simulink model "npc_controller"  (R2022a)
settings: Solver=FixedStepDiscrete  StartTime=0.0  StopTime=20  RelTol=1e-3  EnableMultiTasking=on
undefined symbols (not defined in the file): CAN_O_INT, CANA_BASE, Down, GPTRIP1SEL, GPTRIP2SEL, GPTRIP3SEL, Tsw, TZ1, TZ2, TZ3, Up
libraries: simulink x147, hdlsllib x90, c2802xlib x34, c2837xDlib x20, c280xlib x12, canmsglib x9, c2838xlib x8, idelinklib_common x3, c2806xlib x2, slpidlib x2, c28004xlib x2, c281xlib x2
(part 29 of 42)

== system npc_controller/IDLE_AND_TIMER/codegen/IDLE/idle_task/report_status_flag_bits ==
  Action Port : ActionPort  ActionPortLabel=case [ 0 ]:
  Add : Sum  Inputs=+++++++++++++
  Bit Shift1 : hdlsllib/Logic and Bit Operations/Bit Shift  mode=Shift Left Logical  N=4
  Bit Shift10 : hdlsllib/Logic and Bit Operations/Bit Shift  mode=Shift Left Logical  N=13
  Bit Shift11 : hdlsllib/Logic and Bit Operations/Bit Shift  mode=Shift Left Logical  N=14
  Bit Shift12 : hdlsllib/Logic and Bit Operations/Bit Shift  mode=Shift Left Logical  N=15
  Bit Shift2 : hdlsllib/Logic and Bit Operations/Bit Shift  mode=Shift Left Logical  N=5
  Bit Shift3 : hdlsllib/Logic and Bit Operations/Bit Shift  mode=Shift Left Logical  N=6
  Bit Shift4 : hdlsllib/Logic and Bit Operations/Bit Shift  mode=Shift Left Logical  N=8
  Bit Shift5 : hdlsllib/Logic and Bit Operations/Bit Shift  mode=Shift Left Logical  N=9
  Bit Shift6 : hdlsllib/Logic and Bit Operations/Bit Shift  mode=Shift Left Logical  N=7
  Bit Shift7 : hdlsllib/Logic and Bit Operations/Bit Shift  mode=Shift Left Logical  N=10
  Bit Shift8 : hdlsllib/Logic and Bit Operations/Bit Shift  mode=Shift Left Logical  N=11
  Bit Shift9 : hdlsllib/Logic and Bit Operations/Bit Shift  mode=Shift Left Logical  N=12
  Data Store Read1 : DataStoreRead  DataStoreName=pos_seq  IndexOptions=Index vector (dialog)  Indices=1  OutputSizes=1
  Data Store Read10 : DataStoreRead  DataStoreName=pfc_en  IndexOptions=Index vector (dialog)  Indices=1  OutputSizes=1
  Data Store Read12 : DataStoreRead  DataStoreName=rec_en  IndexOptions=Index vector (dialog)  Indices=1  OutputSizes=1
  Data Store Read13 : DataStoreRead  DataStoreName=ac_ok  IndexOptions=Index vector (dialog)  Indices=1  OutputSizes=1
  Data Store Read14 : DataStoreRead  DataStoreName=can_on_cmd  IndexOptions=Index vector (dialog)  Indices=1  OutputSizes=1
  Data Store Read2 : DataStoreRead  DataStoreName=clllc_ok  IndexOptions=Index vector (dialog)  Indices=1  OutputSizes=1
  Data Store Read3 : DataStoreRead  DataStoreName=npc_fault  IndexOptions=Index vector (dialog)  Indices=1  OutputSizes=1
  Data Store Read4 : DataStoreRead  DataStoreName=inv_en  IndexOptions=Index vector (dialog)  Indices=1  OutputSizes=1
  Data Store Read5 : DataStoreRead  DataStoreName=pfc_ok  IndexOptions=Index vector (dialog)  Indices=1  OutputSizes=1
  Data Store Read6 : DataStoreRead  DataStoreName=state_control  IndexOptions=Index vector (dialog)  Indices=1  OutputSizes=1
  Data Store Read7 : DataStoreRead  DataStoreName=relay_ctrl  IndexOptions=Index vector (dialog)  Indices=1  OutputSizes=1
  Data Store Read8 : DataStoreRead  DataStoreName=ot_fault  IndexOptions=Index vector (dialog)  Indices=1  OutputSizes=1
  Data Store Read9 : DataStoreRead  DataStoreName=can_timeout  IndexOptions=Index vector (dialog)  Indices=1  OutputSizes=1
  Data Store Write : DataStoreWrite  DataStoreName=sPriStatus  IndexOptions=Index vector (dialog)  Indices=1  OutputSizes=1
  Data Store Write4 : DataStoreWrite  Commented=on  DataStoreName=u8ThermalFlags  IndexOptions=Index vector (dialog)  Indices=1  OutputSizes=1
  Data Store Write5 : DataStoreWrite  Commented=on  DataStoreName=u8Reserved1  IndexOptions=Index vector (dialog)  Indices=1  OutputSizes=1
  Data Store Write6 : DataStoreWrite  Commented=on  DataStoreName=u16Reserved1  IndexOptions=Index vector (dialog)  Indices=1  OutputSizes=1
  Data Type Conversion{,1..12} (13 alike) : DataTypeConversion  OutDataTypeStr=uint16  SaturateOnIntegerOverflow=off  RndMeth=Floor
  wires:
  Bit Shift9/1 -> Add/10
  Data Store Read8/1 -> Data Type Conversion11/1
  Data Type Conversion10/1 -> Bit Shift10/1
  Data Type Conversion2/1 -> Bit Shift2/1
  Data Store Read1/1 -> Data Type Conversion5/1
  Bit Shift5/1 -> Add/7
  Data Type Conversion9/1 -> Bit Shift9/1
  Data Type Conversion12/1 -> Bit Shift12/1
  Data Store Read6/1 -> Data Type Conversion/1
  Add/1 -> Data Store Write/1
  Data Store Read9/1 -> Data Type Conversion12/1
  Data Store Read7/1 -> Data Type Conversion6/1
  Bit Shift7/1 -> Add/8
  Data Type Conversion/1 -> Add/1
  Data Type Conversion1/1 -> Bit Shift1/1
  Data Type Conversion8/1 -> Bit Shift8/1
  Bit Shift4/1 -> Add/6
  Data Store Read5/1 -> Data Type Conversion8/1
  Bit Shift3/1 -> Add/4
  Data Type Conversion11/1 -> Bit Shift11/1
  Data Type Conversion3/1 -> Bit Shift3/1
  Bit Shift10/1 -> Add/11
  Bit Shift6/1 -> Add/5
  Bit Shift11/1 -> Add/12
  Bit Shift1/1 -> Add/2
  Data Store Read14/1 -> Data Type Conversion4/1
  Data Store Read3/1 -> Data Type Conversion10/1
  Bit Shift12/1 -> Add/13
  Bit Shift2/1 -> Add/3
  Data Type Conversion5/1 -> Bit Shift4/1
  Data Type Conversion4/1 -> Bit Shift6/1
  Data Store Read10/1 -> Data Type Conversion1/1
  Data Type Conversion6/1 -> Bit Shift5/1
  Data Store Read13/1 -> Data Type Conversion7/1
  Bit Shift8/1 -> Add/9
  Data Store Read2/1 -> Data Type Conversion9/1
  Data Store Read4/1 -> Data Type Conversion3/1
  Data Store Read12/1 -> Data Type Conversion2/1
  Data Type Conversion7/1 -> Bit Shift7/1

== system npc_controller/IDLE_AND_TIMER/codegen/IDLE/idle_task/set_tmp_mux ==
  Action Port : ActionPort  ActionPortLabel=case [ 4 ]:
  Function-Call Generator : simulink/Ports & Subsystems/Function-Call Generator  sample_time=-1  numberOfIterations=1  DisallowWideOutput=off
  Function-Call Split : FunctionCallSplit  NumOutputPorts=2
  Function-Call Split1 : FunctionCallSplit  NumOutputPorts=2
  incr_cnt_tmp_mux : Subsystem  TreatAsAtomicUnit=on
      settings: RTWSystemCode=Inline
  parse_cnt_tmp_mux : Subsystem  TreatAsAtomicUnit=on
      settings: RTWSystemCode=Inline
  set_tmp_mux : Subsystem
  wires:
  Function-Call Generator/1 -> Function-Call Split/1
  Function-Call Split/1 -> parse_cnt_tmp_mux/Trigger
  Function-Call Split1/2 -> incr_cnt_tmp_mux/Trigger
  Function-Call Split1/1 -> set_tmp_mux/Trigger
  Function-Call Split/2 -> Function-Call Split1/1

== system npc_controller/IDLE_AND_TIMER/codegen/IDLE/idle_task/watchdog ==
  note: Note add MLE
  Action Port : ActionPort  ActionPortLabel=case [ 1 ]:
  Watchdog : c281xlib/Watchdog  resetsrc=Specify via dialog  sample=-1
      settings: SourceProductBaseCode=TIC2000

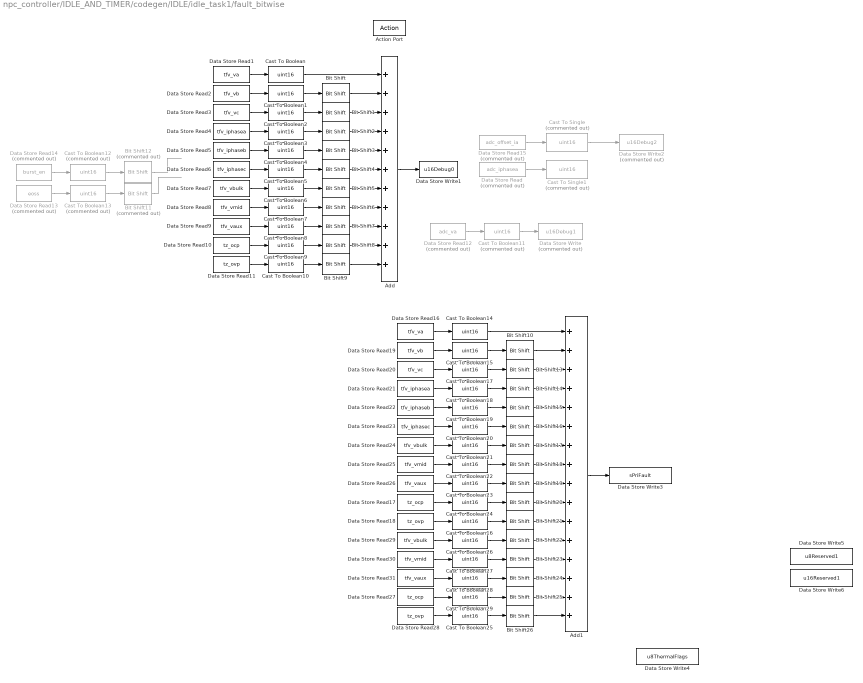
== system npc_controller/IDLE_AND_TIMER/codegen/IDLE/idle_task1/fault_bitwise ==
  Action Port : ActionPort  ActionPortLabel=case [ 5 ]:
  Add : Sum  Inputs=+++++++++++
  Add1 : Sum  Inputs=++++++++++++++++
  Bit Shift : hdlsllib/Logic and Bit Operations/Bit Shift  mode=Shift Left Logical  N=1
  Bit Shift1 : hdlsllib/Logic and Bit Operations/Bit Shift  mode=Shift Left Logical  N=2
  Bit Shift10 : hdlsllib/Logic and Bit Operations/Bit Shift  mode=Shift Left Logical  N=1
  Bit Shift11 : hdlsllib/Logic and Bit Operations/Bit Shift  Commented=on  mode=Shift Left Logical  N=11
  Bit Shift12 : hdlsllib/Logic and Bit Operations/Bit Shift  Commented=on  mode=Shift Left Logical  N=10
  Bit Shift13 : hdlsllib/Logic and Bit Operations/Bit Shift  mode=Shift Left Logical  N=2
  Bit Shift14 : hdlsllib/Logic and Bit Operations/Bit Shift  mode=Shift Left Logical  N=3
  Bit Shift15 : hdlsllib/Logic and Bit Operations/Bit Shift  mode=Shift Left Logical  N=4
  Bit Shift16 : hdlsllib/Logic and Bit Operations/Bit Shift  mode=Shift Left Logical  N=5
  Bit Shift17 : hdlsllib/Logic and Bit Operations/Bit Shift  mode=Shift Left Logical  N=6
  Bit Shift18 : hdlsllib/Logic and Bit Operations/Bit Shift  mode=Shift Left Logical  N=7
  Bit Shift19 : hdlsllib/Logic and Bit Operations/Bit Shift  mode=Shift Left Logical  N=8
  Bit Shift2 : hdlsllib/Logic and Bit Operations/Bit Shift  mode=Shift Left Logical  N=3
  Bit Shift20 : hdlsllib/Logic and Bit Operations/Bit Shift  mode=Shift Left Logical  N=9
  Bit Shift21 : hdlsllib/Logic and Bit Operations/Bit Shift  mode=Shift Left Logical  N=10
  Bit Shift22 : hdlsllib/Logic and Bit Operations/Bit Shift  mode=Shift Left Logical  N=11
  Bit Shift23 : hdlsllib/Logic and Bit Operations/Bit Shift  mode=Shift Left Logical  N=12
  Bit Shift24 : hdlsllib/Logic and Bit Operations/Bit Shift  mode=Shift Left Logical  N=13
  Bit Shift25 : hdlsllib/Logic and Bit Operations/Bit Shift  mode=Shift Left Logical  N=14
  Bit Shift26 : hdlsllib/Logic and Bit Operations/Bit Shift  mode=Shift Left Logical  N=15
  Bit Shift3 : hdlsllib/Logic and Bit Operations/Bit Shift  mode=Shift Left Logical  N=4
  Bit Shift4 : hdlsllib/Logic and Bit Operations/Bit Shift  mode=Shift Left Logical  N=5
  Bit Shift5 : hdlsllib/Logic and Bit Operations/Bit Shift  mode=Shift Left Logical  N=6
  Bit Shift6 : hdlsllib/Logic and Bit Operations/Bit Shift  mode=Shift Left Logical  N=7
  Bit Shift7 : hdlsllib/Logic and Bit Operations/Bit Shift  mode=Shift Left Logical  N=8
  Bit Shift8 : hdlsllib/Logic and Bit Operations/Bit Shift  mode=Shift Left Logical  N=9
  Bit Shift9 : hdlsllib/Logic and Bit Operations/Bit Shift  mode=Shift Left Logical  N=10
  Cast To Boolean{,1..10,14..29} (27 alike) : DataTypeConversion  OutDataTypeStr=uint16  SaturateOnIntegerOverflow=off  RndMeth=Floor
  Cast To Boolean11 : DataTypeConversion  Commented=on  OutDataTypeStr=uint16  SaturateOnIntegerOverflow=off  RndMeth=Floor
  Cast To Boolean12 : DataTypeConversion  Commented=on  OutDataTypeStr=uint16  SaturateOnIntegerOverflow=off  RndMeth=Floor
  Cast To Boolean13 : DataTypeConversion  Commented=on  OutDataTypeStr=uint16  SaturateOnIntegerOverflow=off  RndMeth=Floor
  Cast To Single : DataTypeConversion  Commented=on  OutDataTypeStr=uint16  SaturateOnIntegerOverflow=off  RndMeth=Floor
  Cast To Single1 : DataTypeConversion  Commented=on  OutDataTypeStr=uint16  SaturateOnIntegerOverflow=off  RndMeth=Floor
  Data Store Read : DataStoreRead  Commented=on  DataStoreName=adc_iphasea  IndexOptions=Index vector (dialog)  Indices=1  OutputSizes=1
  Data Store Read1 : DataStoreRead  DataStoreName=tfv_va  IndexOptions=Index vector (dialog)  Indices=1  OutputSizes=1
  Data Store Read10 : DataStoreRead  DataStoreName=tz_ocp  IndexOptions=Index vector (dialog)  Indices=1  OutputSizes=1
  Data Store Read11 : DataStoreRead  DataStoreName=tz_ovp  IndexOptions=Index vector (dialog)  Indices=1  OutputSizes=1
  Data Store Read12 : DataStoreRead  Commented=on  DataStoreName=adc_va  IndexOptions=Index vector (dialog)  Indices=1  OutputSizes=1
  Data Store Read13 : DataStoreRead  Commented=on  DataStoreName=eoss  IndexOptions=Index vector (dialog)  Indices=1  OutputSizes=1
  Data Store Read14 : DataStoreRead  Commented=on  DataStoreName=burst_en  IndexOptions=Index vector (dialog)  Indices=1  OutputSizes=1
  Data Store Read15 : DataStoreRead  Commented=on  DataStoreName=adc_offset_ia  IndexOptions=Index vector (dialog)  Indices=1  OutputSizes=1
  Data Store Read16 : DataStoreRead  DataStoreName=tfv_va  IndexOptions=Index vector (dialog)  Indices=1  OutputSizes=1
  Data Store Read17 : DataStoreRead  DataStoreName=tz_ocp  IndexOptions=Index vector (dialog)  Indices=1  OutputSizes=1
  Data Store Read18 : DataStoreRead  DataStoreName=tz_ovp  IndexOptions=Index vector (dialog)  Indices=1  OutputSizes=1
  Data Store Read19 : DataStoreRead  DataStoreName=tfv_vb  IndexOptions=Index vector (dialog)  Indices=1  OutputSizes=1
  Data Store Read2 : DataStoreRead  DataStoreName=tfv_vb  IndexOptions=Index vector (dialog)  Indices=1  OutputSizes=1
  Data Store Read20 : DataStoreRead  DataStoreName=tfv_vc  IndexOptions=Index vector (dialog)  Indices=1  OutputSizes=1
  Data Store Read21 : DataStoreRead  DataStoreName=tfv_iphasea  IndexOptions=Index vector (dialog)  Indices=1  OutputSizes=1
  Data Store Read22 : DataStoreRead  DataStoreName=tfv_iphaseb  IndexOptions=Index vector (dialog)  Indices=1  OutputSizes=1
  Data Store Read23 : DataStoreRead  DataStoreName=tfv_iphasec  IndexOptions=Index vector (dialog)  Indices=1  OutputSizes=1
  Data Store Read24 : DataStoreRead  DataStoreName=tfv_vbulk  IndexOptions=Index vector (dialog)  Indices=1  OutputSizes=1
  Data Store Read25 : DataStoreRead  DataStoreName=tfv_vmid  IndexOptions=Index vector (dialog)  Indices=1  OutputSizes=1
  Data Store Read26 : DataStoreRead  DataStoreName=tfv_vaux  IndexOptions=Index vector (dialog)  Indices=1  OutputSizes=1
  Data Store Read27 : DataStoreRead  DataStoreName=tz_ocp  IndexOptions=Index vector (dialog)  Indices=1  OutputSizes=1
  Data Store Read28 : DataStoreRead  DataStoreName=tz_ovp  IndexOptions=Index vector (dialog)  Indices=1  OutputSizes=1
  Data Store Read29 : DataStoreRead  DataStoreName=tfv_vbulk  IndexOptions=Index vector (dialog)  Indices=1  OutputSizes=1
  Data Store Read3 : DataStoreRead  DataStoreName=tfv_vc  IndexOptions=Index vector (dialog)  Indices=1  OutputSizes=1
  Data Store Read30 : DataStoreRead  DataStoreName=tfv_vmid  IndexOptions=Index vector (dialog)  Indices=1  OutputSizes=1
  Data Store Read31 : DataStoreRead  DataStoreName=tfv_vaux  IndexOptions=Index vector (dialog)  Indices=1  OutputSizes=1
  Data Store Read4 : DataStoreRead  DataStoreName=tfv_iphasea  IndexOptions=Index vector (dialog)  Indices=1  OutputSizes=1
  Data Store Read5 : DataStoreRead  DataStoreName=tfv_iphaseb  IndexOptions=Index vector (dialog)  Indices=1  OutputSizes=1
  Data Store Read6 : DataStoreRead  DataStoreName=tfv_iphasec  IndexOptions=Index vector (dialog)  Indices=1  OutputSizes=1
  Data Store Read7 : DataStoreRead  DataStoreName=tfv_vbulk  IndexOptions=Index vector (dialog)  Indices=1  OutputSizes=1
  Data Store Read8 : DataStoreRead  DataStoreName=tfv_vmid  IndexOptions=Index vector (dialog)  Indices=1  OutputSizes=1
  Data Store Read9 : DataStoreRead  DataStoreName=tfv_vaux  IndexOptions=Index vector (dialog)  Indices=1  OutputSizes=1
  Data Store Write : DataStoreWrite  Commented=on  DataStoreName=u16Debug1  IndexOptions=Index vector (dialog)  Indices=1  OutputSizes=1
  Data Store Write1 : DataStoreWrite  DataStoreName=u16Debug0  IndexOptions=Index vector (dialog)  Indices=1  OutputSizes=1
  Data Store Write2 : DataStoreWrite  Commented=on  DataStoreName=u16Debug2  IndexOptions=Index vector (dialog)  Indices=1  OutputSizes=1
  Data Store Write3 : DataStoreWrite  DataStoreName=sPriFault  IndexOptions=Index vector (dialog)  Indices=1  OutputSizes=1
  Data Store Write4 : DataStoreWrite  DataStoreName=u8ThermalFlags  IndexOptions=Index vector (dialog)  Indices=1  OutputSizes=1
  Data Store Write5 : DataStoreWrite  DataStoreName=u8Reserved1  IndexOptions=Index vector (dialog)  Indices=1  OutputSizes=1
  Data Store Write6 : DataStoreWrite  DataStoreName=u16Reserved1  IndexOptions=Index vector (dialog)  Indices=1  OutputSizes=1
  wires:
  Add/1 -> Data Store Write1/1
  Data Store Read7/1 -> Cast To Boolean6/1
  Cast To Boolean7/1 -> Bit Shift6/1
  Data Store Read3/1 -> Cast To Boolean2/1
  Cast To Boolean2/1 -> Bit Shift1/1
  Data Store Read1/1 -> Cast To Boolean/1
  Bit Shift5/1 -> Add/7
  Bit Shift/1 -> Add/2
  Data Store Read8/1 -> Cast To Boolean7/1
  Bit Shift3/1 -> Add/5
  Cast To Boolean6/1 -> Bit Shift5/1
  Data Store Read2/1 -> Cast To Boolean1/1
  Bit Shift4/1 -> Add/6
  Bit Shift2/1 -> Add/4
  Cast To Boolean5/1 -> Bit Shift4/1
  Cast To Boolean/1 -> Add/1
  Cast To Boolean1/1 -> Bit Shift/1
  Bit Shift6/1 -> Add/8
  Cast To Boolean3/1 -> Bit Shift2/1
  Cast To Boolean4/1 -> Bit Shift3/1
  Bit Shift1/1 -> Add/3
  Cast To Boolean9/1 -> Bit Shift8/1
  Bit Shift8/1 -> Add/10
  Data Store Read10/1 -> Cast To Boolean9/1
  Data Store Read9/1 -> Cast To Boolean8/1
  Cast To Boolean8/1 -> Bit Shift7/1
  Bit Shift7/1 -> Add/9
  Bit Shift11/1 -> ?
  Bit Shift12/1 -> ?
  Cast To Boolean13/1 -> Bit Shift11/1
  Cast To Boolean12/1 -> Bit Shift12/1
  Data Store Read13/1 -> Cast To Boolean13/1
  Data Store Read14/1 -> Cast To Boolean12/1
  Bit Shift9/1 -> Add/11
  Data Store Read11/1 -> Cast To Boolean10/1
  Cast To Boolean10/1 -> Bit Shift9/1
  Cast To Boolean11/1 -> Data Store Write/1
  Data Store Read12/1 -> Cast To Boolean11/1
  Data Store Read15/1 -> Cast To Single/1
  Data Store Read/1 -> Cast To Single1/1
  Cast To Single/1 -> Data Store Write2/1
  Data Store Read4/1 -> Cast To Boolean3/1
  Data Store Read5/1 -> Cast To Boolean4/1
  Data Store Read6/1 -> Cast To Boolean5/1
  Data Store Read23/1 -> Cast To Boolean20/1
  Data Store Read22/1 -> Cast To Boolean19/1
  Data Store Read21/1 -> Cast To Boolean18/1
  Cast To Boolean16/1 -> Bit Shift21/1
  Data Store Read18/1 -> Cast To Boolean16/1
  Bit Shift21/1 -> Add1/11
  Bit Shift19/1 -> Add1/9
  Cast To Boolean23/1 -> Bit Shift19/1
  Data Store Read26/1 -> Cast To Boolean23/1
  Data Store Read17/1 -> Cast To Boolean24/1
  Bit Shift20/1 -> Add1/10
  Cast To Boolean24/1 -> Bit Shift20/1
  Bit Shift13/1 -> Add1/3
  Cast To Boolean19/1 -> Bit Shift15/1
  Cast To Boolean18/1 -> Bit Shift14/1
  Bit Shift18/1 -> Add1/8
  Cast To Boolean15/1 -> Bit Shift10/1
  Cast To Boolean14/1 -> Add1/1
  Cast To Boolean20/1 -> Bit Shift16/1
  Bit Shift14/1 -> Add1/4
  Bit Shift16/1 -> Add1/6
  Data Store Read19/1 -> Cast To Boolean15/1
  Cast To Boolean21/1 -> Bit Shift17/1
  Bit Shift15/1 -> Add1/5
  Data Store Read25/1 -> Cast To Boolean22/1
  Bit Shift10/1 -> Add1/2
  Bit Shift17/1 -> Add1/7
  Data Store Read16/1 -> Cast To Boolean14/1
  Cast To Boolean17/1 -> Bit Shift13/1
  Data Store Read20/1 -> Cast To Boolean17/1
  Cast To Boolean22/1 -> Bit Shift18/1
  Data Store Read24/1 -> Cast To Boolean21/1
  Data Store Read29/1 -> Cast To Boolean26/1
  Cast To Boolean27/1 -> Bit Shift23/1
  Bit Shift22/1 -> Add1/12
  Data Store Read30/1 -> Cast To Boolean27/1
  Cast To Boolean26/1 -> Bit Shift22/1
  Bit Shift23/1 -> Add1/13
  Cast To Boolean29/1 -> Bit Shift25/1
  Bit Shift25/1 -> Add1/15
  Data Store Read27/1 -> Cast To Boolean29/1
  Data Store Read31/1 -> Cast To Boolean28/1
  Cast To Boolean28/1 -> Bit Shift24/1
  Bit Shift24/1 -> Add1/14
  Bit Shift26/1 -> Add1/16
  Data Store Read28/1 -> Cast To Boolean25/1
  Cast To Boolean25/1 -> Bit Shift26/1
  Add1/1 -> Data Store Write3/1

== system npc_controller/IDLE_AND_TIMER/codegen/IDLE/idle_task1/get_adc_tmp_mux ==
  Action Port : ActionPort  ActionPortLabel=case [ 4 ]:
  Data Store Read : DataStoreRead  DataStoreName=cnt_tmp_mux  IndexOptions=Index vector (dialog)  Indices=1  OutputSizes=1
  Data Store Read1 : DataStoreRead  DataStoreName=adc_temp_mux  IndexOptions=Index vector (dialog)  Indices=1  OutputSizes=1
  Switch Case : SwitchCase  CaseConditions={0, 1, 2, 3}
  get_tmp_mux_inlet : Subsystem  TreatAsAtomicUnit=on
  get_tmp_mux_npca : Subsystem  TreatAsAtomicUnit=on
  get_tmp_mux_npcb : Subsystem  TreatAsAtomicUnit=on
  get_tmp_mux_npcc : Subsystem  TreatAsAtomicUnit=on
  wires:
  Data Store Read/1 -> Switch Case/1
  Switch Case/1 -> get_tmp_mux_npca/Action
  Switch Case/2 -> get_tmp_mux_npcb/Action
  Switch Case/3 -> get_tmp_mux_npcc/Action
  Switch Case/4 -> get_tmp_mux_inlet/Action
  Data Store Read1/1 -> get_tmp_mux_npcb/1(In1), get_tmp_mux_npca/1(In1), get_tmp_mux_npcc/1(In1), get_tmp_mux_inlet/1(In1)

== system npc_controller/IDLE_AND_TIMER/codegen/IDLE/idle_task1/hkeep ==
  note: prot and status
  Action Port : ActionPort  ActionPortLabel=case [ 1 ]:
  Function-Call Generator1 : simulink/Ports & Subsystems/Function-Call Generator  sample_time=-1  numberOfIterations=1  DisallowWideOutput=off
  Function-Call Split3 : FunctionCallSplit  NumOutputPorts=2
  tfv : Subsystem  TreatAsAtomicUnit=on
      settings: RTWSystemCode=Inline
  tz : Subsystem  TreatAsAtomicUnit=on
      settings: RTWSystemCode=Inline
  wires:
  Function-Call Split3/1 -> tz/Trigger
  Function-Call Split3/2 -> tfv/Trigger
  Function-Call Generator1/1 -> Function-Call Split3/1

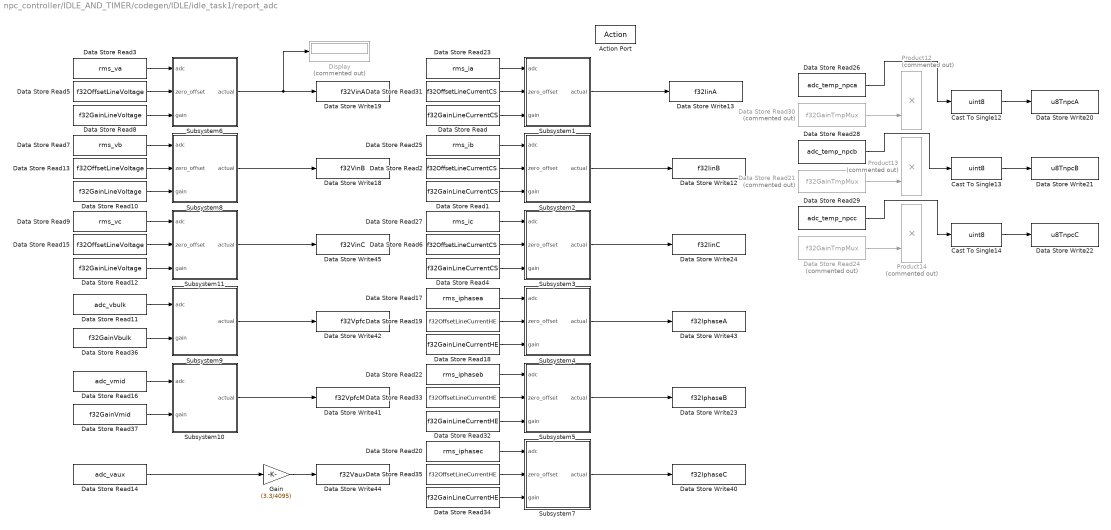
== system npc_controller/IDLE_AND_TIMER/codegen/IDLE/idle_task1/report_adc ==
  Action Port : ActionPort  ActionPortLabel=case [ 2 ]:
  Cast To Single12 : DataTypeConversion  OutDataTypeStr=uint8  SaturateOnIntegerOverflow=off  RndMeth=Floor
  Cast To Single13 : DataTypeConversion  OutDataTypeStr=uint8  SaturateOnIntegerOverflow=off  RndMeth=Floor
  Cast To Single14 : DataTypeConversion  OutDataTypeStr=uint8  SaturateOnIntegerOverflow=off  RndMeth=Floor
  Data Store Read : DataStoreRead  DataStoreName=f32GainLineCurrentCS  IndexOptions=Index vector (dialog)  Indices=1  OutputSizes=1
  Data Store Read1 : DataStoreRead  DataStoreName=f32GainLineCurrentCS  IndexOptions=Index vector (dialog)  Indices=1  OutputSizes=1
  Data Store Read10 : DataStoreRead  DataStoreName=f32GainLineVoltage  IndexOptions=Index vector (dialog)  Indices=1  OutputSizes=1
  Data Store Read11 : DataStoreRead  DataStoreName=adc_vbulk  IndexOptions=Index vector (dialog)  Indices=1  OutputSizes=1
  Data Store Read12 : DataStoreRead  DataStoreName=f32GainLineVoltage  IndexOptions=Index vector (dialog)  Indices=1  OutputSizes=1
  Data Store Read13 : DataStoreRead  DataStoreName=f32OffsetLineVoltage  IndexOptions=Index vector (dialog)  Indices=1  OutputSizes=1
  Data Store Read14 : DataStoreRead  DataStoreName=adc_vaux  IndexOptions=Index vector (dialog)  Indices=1  OutputSizes=1
  Data Store Read15 : DataStoreRead  DataStoreName=f32OffsetLineVoltage  IndexOptions=Index vector (dialog)  Indices=1  OutputSizes=1
  Data Store Read16 : DataStoreRead  DataStoreName=adc_vmid  IndexOptions=Index vector (dialog)  Indices=1  OutputSizes=1
  Data Store Read17 : DataStoreRead  DataStoreName=rms_iphasea  IndexOptions=Index vector (dialog)  Indices=1  OutputSizes=1
  Data Store Read18 : DataStoreRead  DataStoreName=f32GainLineCurrentHE  IndexOptions=Index vector (dialog)  Indices=1  OutputSizes=1
  Data Store Read19 : DataStoreRead  DataStoreName=f32OffsetLineCurrentHE  IndexOptions=Index vector (dialog)  Indices=1  OutputSizes=1
  Data Store Read2 : DataStoreRead  DataStoreName=f32OffsetLineCurrentCS  IndexOptions=Index vector (dialog)  Indices=1  OutputSizes=1
  Data Store Read20 : DataStoreRead  DataStoreName=rms_iphasec  IndexOptions=Index vector (dialog)  Indices=1  OutputSizes=1
  Data Store Read21 : DataStoreRead  Commented=on  DataStoreName=f32GainTmpMux  IndexOptions=Index vector (dialog)  Indices=1  OutputSizes=1
  Data Store Read22 : DataStoreRead  DataStoreName=rms_iphaseb  IndexOptions=Index vector (dialog)  Indices=1  OutputSizes=1
  Data Store Read23 : DataStoreRead  DataStoreName=rms_ia  IndexOptions=Index vector (dialog)  Indices=1  OutputSizes=1
  Data Store Read24 : DataStoreRead  Commented=on  DataStoreName=f32GainTmpMux  IndexOptions=Index vector (dialog)  Indices=1  OutputSizes=1
  Data Store Read25 : DataStoreRead  DataStoreName=rms_ib  IndexOptions=Index vector (dialog)  Indices=1  OutputSizes=1
  Data Store Read26 : DataStoreRead  DataStoreName=adc_temp_npca  IndexOptions=Index vector (dialog)  Indices=1  OutputSizes=1
  Data Store Read27 : DataStoreRead  DataStoreName=rms_ic  IndexOptions=Index vector (dialog)  Indices=1  OutputSizes=1
  Data Store Read28 : DataStoreRead  DataStoreName=adc_temp_npcb  IndexOptions=Index vector (dialog)  Indices=1  OutputSizes=1
  Data Store Read29 : DataStoreRead  DataStoreName=adc_temp_npcc  IndexOptions=Index vector (dialog)  Indices=1  OutputSizes=1
  Data Store Read3 : DataStoreRead  DataStoreName=rms_va  IndexOptions=Index vector (dialog)  Indices=1  OutputSizes=1
  Data Store Read30 : DataStoreRead  Commented=on  DataStoreName=f32GainTmpMux  IndexOptions=Index vector (dialog)  Indices=1  OutputSizes=1
  Data Store Read31 : DataStoreRead  DataStoreName=f32OffsetLineCurrentCS  IndexOptions=Index vector (dialog)  Indices=1  OutputSizes=1
  Data Store Read32 : DataStoreRead  DataStoreName=f32GainLineCurrentHE  IndexOptions=Index vector (dialog)  Indices=1  OutputSizes=1
  Data Store Read33 : DataStoreRead  DataStoreName=f32OffsetLineCurrentHE  IndexOptions=Index vector (dialog)  Indices=1  OutputSizes=1
  Data Store Read34 : DataStoreRead  DataStoreName=f32GainLineCurrentHE  IndexOptions=Index vector (dialog)  Indices=1  OutputSizes=1
  Data Store Read35 : DataStoreRead  DataStoreName=f32OffsetLineCurrentHE  IndexOptions=Index vector (dialog)  Indices=1  OutputSizes=1
  Data Store Read36 : DataStoreRead  DataStoreName=f32GainVbulk  IndexOptions=Index vector (dialog)  Indices=1  OutputSizes=1
  Data Store Read37 : DataStoreRead  DataStoreName=f32GainVmid  IndexOptions=Index vector (dialog)  Indices=1  OutputSizes=1
  Data Store Read4 : DataStoreRead  DataStoreName=f32GainLineCurrentCS  IndexOptions=Index vector (dialog)  Indices=1  OutputSizes=1
  Data Store Read5 : DataStoreRead  DataStoreName=f32OffsetLineVoltage  IndexOptions=Index vector (dialog)  Indices=1  OutputSizes=1
  Data Store Read6 : DataStoreRead  DataStoreName=f32OffsetLineCurrentCS  IndexOptions=Index vector (dialog)  Indices=1  OutputSizes=1
  Data Store Read7 : DataStoreRead  DataStoreName=rms_vb  IndexOptions=Index vector (dialog)  Indices=1  OutputSizes=1
  Data Store Read8 : DataStoreRead  DataStoreName=f32GainLineVoltage  IndexOptions=Index vector (dialog)  Indices=1  OutputSizes=1
  Data Store Read9 : DataStoreRead  DataStoreName=rms_vc  IndexOptions=Index vector (dialog)  Indices=1  OutputSizes=1
  Data Store Write12 : DataStoreWrite  DataStoreName=f32IinB  IndexOptions=Index vector (dialog)  Indices=1  OutputSizes=1
  Data Store Write13 : DataStoreWrite  DataStoreName=f32IinA  IndexOptions=Index vector (dialog)  Indices=1  OutputSizes=1
  Data Store Write18 : DataStoreWrite  DataStoreName=f32VinB  IndexOptions=Index vector (dialog)  Indices=1  OutputSizes=1
  Data Store Write19 : DataStoreWrite  DataStoreName=f32VinA  IndexOptions=Index vector (dialog)  Indices=1  OutputSizes=1
  Data Store Write20 : DataStoreWrite  DataStoreName=u8TnpcA  IndexOptions=Index vector (dialog)  Indices=1  OutputSizes=1
  Data Store Write21 : DataStoreWrite  DataStoreName=u8TnpcB  IndexOptions=Index vector (dialog)  Indices=1  OutputSizes=1
  Data Store Write22 : DataStoreWrite  DataStoreName=u8TnpcC  IndexOptions=Index vector (dialog)  Indices=1  OutputSizes=1
  Data Store Write23 : DataStoreWrite  DataStoreName=f32IphaseB  IndexOptions=Index vector (dialog)  Indices=1  OutputSizes=1
  Data Store Write24 : DataStoreWrite  DataStoreName=f32IinC  IndexOptions=Index vector (dialog)  Indices=1  OutputSizes=1
  Data Store Write40 : DataStoreWrite  DataStoreName=f32IphaseC  IndexOptions=Index vector (dialog)  Indices=1  OutputSizes=1
  Data Store Write41 : DataStoreWrite  DataStoreName=f32VpfcMid  IndexOptions=Index vector (dialog)  Indices=1  OutputSizes=1
  Data Store Write42 : DataStoreWrite  DataStoreName=f32Vpfc  IndexOptions=Index vector (dialog)  Indices=1  OutputSizes=1
  Data Store Write43 : DataStoreWrite  DataStoreName=f32IphaseA  IndexOptions=Index vector (dialog)  Indices=1  OutputSizes=1
  Data Store Write44 : DataStoreWrite  DataStoreName=f32Vaux  IndexOptions=Index vector (dialog)  Indices=1  OutputSizes=1
  Data Store Write45 : DataStoreWrite  DataStoreName=f32VinC  IndexOptions=Index vector (dialog)  Indices=1  OutputSizes=1
  Display : Display  Commented=on
  Gain : Gain  Gain=(3.3/4095)  ParamDataTypeStr=single  OutDataTypeStr=single
  Product12 : Product  Commented=on  OutDataTypeStr=single
  Product13 : Product  Commented=on  OutDataTypeStr=single
  Product14 : Product  Commented=on  OutDataTypeStr=single
  Subsystem1 : Subsystem
  Subsystem10 : Subsystem
  Subsystem11 : Subsystem
  Subsystem2 : Subsystem
  Subsystem3 : Subsystem
  Subsystem4 : Subsystem
  Subsystem5 : Subsystem
  Subsystem6 : Subsystem
  Subsystem7 : Subsystem
  Subsystem8 : Subsystem
  Subsystem9 : Subsystem
  wires:
  Data Store Read14/1 -> Gain/1
  Cast To Single13/1 -> Data Store Write21/1
  Cast To Single14/1 -> Data Store Write22/1
  Cast To Single12/1 -> Data Store Write20/1
  Data Store Read30/1 -> Product12/2
  Data Store Read21/1 -> Product13/2
  Data Store Read24/1 -> Product14/2
  Data Store Read25/1 -> Subsystem2/1(adc)
  Data Store Read27/1 -> Subsystem3/1(adc)
  Data Store Read17/1 -> Subsystem4/1(adc)
  Data Store Read22/1 -> Subsystem5/1(adc)
  Data Store Read20/1 -> Subsystem7/1(adc)
  Data Store Read2/1 -> Subsystem2/2(zero_offset)
  Data Store Read1/1 -> Subsystem2/3(gain)
  Data Store Read6/1 -> Subsystem3/2(zero_offset)
  Data Store Read4/1 -> Subsystem3/3(gain)
  Data Store Read19/1 -> Subsystem4/2(zero_offset)
  Data Store Read18/1 -> Subsystem4/3(gain)
  Data Store Read32/1 -> Subsystem5/3(gain)
  Data Store Read33/1 -> Subsystem5/2(zero_offset)
  Data Store Read35/1 -> Subsystem7/2(zero_offset)
  Data Store Read34/1 -> Subsystem7/3(gain)
  Data Store Read7/1 -> Subsystem8/1(adc)
  Data Store Read9/1 -> Subsystem11/1(adc)
  Data Store Read11/1 -> Subsystem9/1(adc)
  Data Store Read16/1 -> Subsystem10/1(adc)
  Data Store Read15/1 -> Subsystem11/2(zero_offset)
  Data Store Read12/1 -> Subsystem11/3(gain)
  Data Store Read36/1 -> Subsystem9/2(gain)
  Data Store Read37/1 -> Subsystem10/2(gain)
  Gain/1 -> Data Store Write44/1
  Data Store Read5/1 -> Subsystem6/2(zero_offset)
  Data Store Read8/1 -> Subsystem6/3(gain)
  Data Store Read/1 -> Subsystem1/3(gain)
  Data Store Read31/1 -> Subsystem1/2(zero_offset)
  Data Store Read10/1 -> Subsystem8/3(gain)
  Data Store Read13/1 -> Subsystem8/2(zero_offset)
  Data Store Read26/1 -> Cast To Single12/1
  Data Store Read28/1 -> Cast To Single13/1
  Data Store Read29/1 -> Cast To Single14/1
  Subsystem8/1(actual) -> Data Store Write18/1
  Subsystem11/1(actual) -> Data Store Write45/1
  Subsystem10/1(actual) -> Data Store Write41/1
  Subsystem1/1(actual) -> Data Store Write13/1
  Subsystem2/1(actual) -> Data Store Write12/1
  Data Store Read23/1 -> Subsystem1/1(adc)
  Subsystem9/1(actual) -> Data Store Write42/1
  Subsystem3/1(actual) -> Data Store Write24/1
  Subsystem4/1(actual) -> Data Store Write43/1
  Subsystem5/1(actual) -> Data Store Write23/1
  Subsystem7/1(actual) -> Data Store Write40/1
  Subsystem6/1(actual) -> Display/1, Data Store Write19/1
  Data Store Read3/1 -> Subsystem6/1(adc)

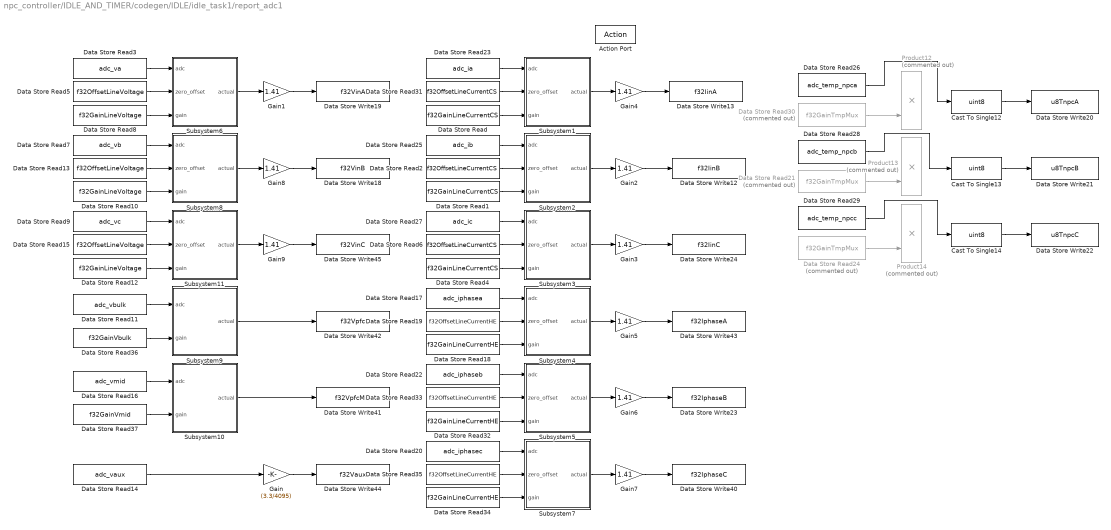
== system npc_controller/IDLE_AND_TIMER/codegen/IDLE/idle_task1/report_adc1 ==
  Action Port : ActionPort
  Cast To Single12 : DataTypeConversion  OutDataTypeStr=uint8  SaturateOnIntegerOverflow=off  RndMeth=Floor
  Cast To Single13 : DataTypeConversion  OutDataTypeStr=uint8  SaturateOnIntegerOverflow=off  RndMeth=Floor
  Cast To Single14 : DataTypeConversion  OutDataTypeStr=uint8  SaturateOnIntegerOverflow=off  RndMeth=Floor
  Data Store Read : DataStoreRead  DataStoreName=f32GainLineCurrentCS  IndexOptions=Index vector (dialog)  Indices=1  OutputSizes=1
  Data Store Read1 : DataStoreRead  DataStoreName=f32GainLineCurrentCS  IndexOptions=Index vector (dialog)  Indices=1  OutputSizes=1
  Data Store Read10 : DataStoreRead  DataStoreName=f32GainLineVoltage  IndexOptions=Index vector (dialog)  Indices=1  OutputSizes=1
  Data Store Read11 : DataStoreRead  DataStoreName=adc_vbulk  IndexOptions=Index vector (dialog)  Indices=1  OutputSizes=1
  Data Store Read12 : DataStoreRead  DataStoreName=f32GainLineVoltage  IndexOptions=Index vector (dialog)  Indices=1  OutputSizes=1
  Data Store Read13 : DataStoreRead  DataStoreName=f32OffsetLineVoltage  IndexOptions=Index vector (dialog)  Indices=1  OutputSizes=1
  Data Store Read14 : DataStoreRead  DataStoreName=adc_vaux  IndexOptions=Index vector (dialog)  Indices=1  OutputSizes=1
  Data Store Read15 : DataStoreRead  DataStoreName=f32OffsetLineVoltage  IndexOptions=Index vector (dialog)  Indices=1  OutputSizes=1
  Data Store Read16 : DataStoreRead  DataStoreName=adc_vmid  IndexOptions=Index vector (dialog)  Indices=1  OutputSizes=1
  Data Store Read17 : DataStoreRead  DataStoreName=adc_iphasea  IndexOptions=Index vector (dialog)  Indices=1  OutputSizes=1
  Data Store Read18 : DataStoreRead  DataStoreName=f32GainLineCurrentHE  IndexOptions=Index vector (dialog)  Indices=1  OutputSizes=1
  Data Store Read19 : DataStoreRead  DataStoreName=f32OffsetLineCurrentHE  IndexOptions=Index vector (dialog)  Indices=1  OutputSizes=1
  Data Store Read2 : DataStoreRead  DataStoreName=f32OffsetLineCurrentCS  IndexOptions=Index vector (dialog)  Indices=1  OutputSizes=1
  Data Store Read20 : DataStoreRead  DataStoreName=adc_iphasec  IndexOptions=Index vector (dialog)  Indices=1  OutputSizes=1
  Data Store Read21 : DataStoreRead  Commented=on  DataStoreName=f32GainTmpMux  IndexOptions=Index vector (dialog)  Indices=1  OutputSizes=1
  Data Store Read22 : DataStoreRead  DataStoreName=adc_iphaseb  IndexOptions=Index vector (dialog)  Indices=1  OutputSizes=1
  Data Store Read23 : DataStoreRead  DataStoreName=adc_ia  IndexOptions=Index vector (dialog)  Indices=1  OutputSizes=1
  Data Store Read24 : DataStoreRead  Commented=on  DataStoreName=f32GainTmpMux  IndexOptions=Index vector (dialog)  Indices=1  OutputSizes=1
  Data Store Read25 : DataStoreRead  DataStoreName=adc_ib  IndexOptions=Index vector (dialog)  Indices=1  OutputSizes=1
  Data Store Read26 : DataStoreRead  DataStoreName=adc_temp_npca  IndexOptions=Index vector (dialog)  Indices=1  OutputSizes=1
  Data Store Read27 : DataStoreRead  DataStoreName=adc_ic  IndexOptions=Index vector (dialog)  Indices=1  OutputSizes=1
  Data Store Read28 : DataStoreRead  DataStoreName=adc_temp_npcb  IndexOptions=Index vector (dialog)  Indices=1  OutputSizes=1
  Data Store Read29 : DataStoreRead  DataStoreName=adc_temp_npcc  IndexOptions=Index vector (dialog)  Indices=1  OutputSizes=1
  Data Store Read3 : DataStoreRead  DataStoreName=adc_va  IndexOptions=Index vector (dialog)  Indices=1  OutputSizes=1
  Data Store Read30 : DataStoreRead  Commented=on  DataStoreName=f32GainTmpMux  IndexOptions=Index vector (dialog)  Indices=1  OutputSizes=1
  Data Store Read31 : DataStoreRead  DataStoreName=f32OffsetLineCurrentCS  IndexOptions=Index vector (dialog)  Indices=1  OutputSizes=1
  Data Store Read32 : DataStoreRead  DataStoreName=f32GainLineCurrentHE  IndexOptions=Index vector (dialog)  Indices=1  OutputSizes=1
  Data Store Read33 : DataStoreRead  DataStoreName=f32OffsetLineCurrentHE  IndexOptions=Index vector (dialog)  Indices=1  OutputSizes=1
  Data Store Read34 : DataStoreRead  DataStoreName=f32GainLineCurrentHE  IndexOptions=Index vector (dialog)  Indices=1  OutputSizes=1
  Data Store Read35 : DataStoreRead  DataStoreName=f32OffsetLineCurrentHE  IndexOptions=Index vector (dialog)  Indices=1  OutputSizes=1
  Data Store Read36 : DataStoreRead  DataStoreName=f32GainVbulk  IndexOptions=Index vector (dialog)  Indices=1  OutputSizes=1
  Data Store Read37 : DataStoreRead  DataStoreName=f32GainVmid  IndexOptions=Index vector (dialog)  Indices=1  OutputSizes=1
  Data Store Read4 : DataStoreRead  DataStoreName=f32GainLineCurrentCS  IndexOptions=Index vector (dialog)  Indices=1  OutputSizes=1
  Data Store Read5 : DataStoreRead  DataStoreName=f32OffsetLineVoltage  IndexOptions=Index vector (dialog)  Indices=1  OutputSizes=1
  Data Store Read6 : DataStoreRead  DataStoreName=f32OffsetLineCurrentCS  IndexOptions=Index vector (dialog)  Indices=1  OutputSizes=1
  Data Store Read7 : DataStoreRead  DataStoreName=adc_vb  IndexOptions=Index vector (dialog)  Indices=1  OutputSizes=1
  Data Store Read8 : DataStoreRead  DataStoreName=f32GainLineVoltage  IndexOptions=Index vector (dialog)  Indices=1  OutputSizes=1
  Data Store Read9 : DataStoreRead  DataStoreName=adc_vc  IndexOptions=Index vector (dialog)  Indices=1  OutputSizes=1
  Data Store Write12 : DataStoreWrite  DataStoreName=f32IinB  IndexOptions=Index vector (dialog)  Indices=1  OutputSizes=1
  Data Store Write13 : DataStoreWrite  DataStoreName=f32IinA  IndexOptions=Index vector (dialog)  Indices=1  OutputSizes=1
  Data Store Write18 : DataStoreWrite  DataStoreName=f32VinB  IndexOptions=Index vector (dialog)  Indices=1  OutputSizes=1
  Data Store Write19 : DataStoreWrite  DataStoreName=f32VinA  IndexOptions=Index vector (dialog)  Indices=1  OutputSizes=1
  Data Store Write20 : DataStoreWrite  DataStoreName=u8TnpcA  IndexOptions=Index vector (dialog)  Indices=1  OutputSizes=1
  Data Store Write21 : DataStoreWrite  DataStoreName=u8TnpcB  IndexOptions=Index vector (dialog)  Indices=1  OutputSizes=1
  Data Store Write22 : DataStoreWrite  DataStoreName=u8TnpcC  IndexOptions=Index vector (dialog)  Indices=1  OutputSizes=1
  Data Store Write23 : DataStoreWrite  DataStoreName=f32IphaseB  IndexOptions=Index vector (dialog)  Indices=1  OutputSizes=1
  Data Store Write24 : DataStoreWrite  DataStoreName=f32IinC  IndexOptions=Index vector (dialog)  Indices=1  OutputSizes=1
  Data Store Write40 : DataStoreWrite  DataStoreName=f32IphaseC  IndexOptions=Index vector (dialog)  Indices=1  OutputSizes=1
  Data Store Write41 : DataStoreWrite  DataStoreName=f32VpfcMid  IndexOptions=Index vector (dialog)  Indices=1  OutputSizes=1
  Data Store Write42 : DataStoreWrite  DataStoreName=f32Vpfc  IndexOptions=Index vector (dialog)  Indices=1  OutputSizes=1
  Data Store Write43 : DataStoreWrite  DataStoreName=f32IphaseA  IndexOptions=Index vector (dialog)  Indices=1  OutputSizes=1
  Data Store Write44 : DataStoreWrite  DataStoreName=f32Vaux  IndexOptions=Index vector (dialog)  Indices=1  OutputSizes=1
  Data Store Write45 : DataStoreWrite  DataStoreName=f32VinC  IndexOptions=Index vector (dialog)  Indices=1  OutputSizes=1
  Gain : Gain  Gain=(3.3/4095)  ParamDataTypeStr=single  OutDataTypeStr=single
  Gain{1..9} (9 alike) : Gain  Gain=1.41  ParamDataTypeStr=single  OutDataTypeStr=single
  Product12 : Product  Commented=on  OutDataTypeStr=single
  Product13 : Product  Commented=on  OutDataTypeStr=single
  Product14 : Product  Commented=on  OutDataTypeStr=single
  Subsystem1 : Subsystem
  Subsystem10 : Subsystem
  Subsystem11 : Subsystem
  Subsystem2 : Subsystem
  Subsystem3 : Subsystem
  Subsystem4 : Subsystem
  Subsystem5 : Subsystem
  Subsystem6 : Subsystem
  Subsystem7 : Subsystem
  Subsystem8 : Subsystem
  Subsystem9 : Subsystem
  wires:
  Data Store Read3/1 -> Subsystem6/1(adc)
  Subsystem8/1(actual) -> Gain8/1
  Subsystem11/1(actual) -> Gain9/1
  Subsystem5/1(actual) -> Gain6/1
  Subsystem7/1(actual) -> Gain7/1
  Subsystem4/1(actual) -> Gain5/1
  Subsystem3/1(actual) -> Gain3/1
  Subsystem2/1(actual) -> Gain2/1
  Gain7/1 -> Data Store Write40/1
  Gain6/1 -> Data Store Write23/1
  Gain5/1 -> Data Store Write43/1
  Gain3/1 -> Data Store Write24/1
  Subsystem9/1(actual) -> Data Store Write42/1
  Data Store Read23/1 -> Subsystem1/1(adc)
  Gain1/1 -> Data Store Write19/1
  Subsystem6/1(actual) -> Gain1/1
  Gain2/1 -> Data Store Write12/1
  Gain4/1 -> Data Store Write13/1
  Subsystem10/1(actual) -> Data Store Write41/1
  Gain9/1 -> Data Store Write45/1
  Gain8/1 -> Data Store Write18/1
  Data Store Read29/1 -> Cast To Single14/1
  Data Store Read28/1 -> Cast To Single13/1
  Data Store Read26/1 -> Cast To Single12/1
  Data Store Read13/1 -> Subsystem8/2(zero_offset)
  Data Store Read10/1 -> Subsystem8/3(gain)
  Data Store Read31/1 -> Subsystem1/2(zero_offset)
  Data Store Read/1 -> Subsystem1/3(gain)
  Data Store Read8/1 -> Subsystem6/3(gain)
  Data Store Read5/1 -> Subsystem6/2(zero_offset)
  Gain/1 -> Data Store Write44/1
  Data Store Read37/1 -> Subsystem10/2(gain)
  Data Store Read36/1 -> Subsystem9/2(gain)
  Data Store Read12/1 -> Subsystem11/3(gain)
  Data Store Read15/1 -> Subsystem11/2(zero_offset)
  Data Store Read16/1 -> Subsystem10/1(adc)
  Data Store Read11/1 -> Subsystem9/1(adc)
  Data Store Read9/1 -> Subsystem11/1(adc)
  Data Store Read7/1 -> Subsystem8/1(adc)
  Data Store Read34/1 -> Subsystem7/3(gain)
  Data Store Read35/1 -> Subsystem7/2(zero_offset)
  Data Store Read33/1 -> Subsystem5/2(zero_offset)
  Data Store Read32/1 -> Subsystem5/3(gain)
  Data Store Read18/1 -> Subsystem4/3(gain)
  Data Store Read19/1 -> Subsystem4/2(zero_offset)
  Data Store Read4/1 -> Subsystem3/3(gain)
  Data Store Read6/1 -> Subsystem3/2(zero_offset)
  Data Store Read1/1 -> Subsystem2/3(gain)
  Data Store Read2/1 -> Subsystem2/2(zero_offset)
  Data Store Read20/1 -> Subsystem7/1(adc)
  Data Store Read22/1 -> Subsystem5/1(adc)
  Data Store Read17/1 -> Subsystem4/1(adc)
  Data Store Read27/1 -> Subsystem3/1(adc)
  Data Store Read25/1 -> Subsystem2/1(adc)
  Subsystem1/1(actual) -> Gain4/1
  Data Store Read24/1 -> Product14/2
  Data Store Read21/1 -> Product13/2
  Data Store Read30/1 -> Product12/2
  Cast To Single12/1 -> Data Store Write20/1
  Cast To Single14/1 -> Data Store Write22/1
  Cast To Single13/1 -> Data Store Write21/1
  Data Store Read14/1 -> Gain/1

== system npc_controller/IDLE_AND_TIMER/codegen/IDLE/idle_task1/set_tmp_mux ==
  Action Port : ActionPort  ActionPortLabel=case [ 3 ]:
  Function-Call Generator : simulink/Ports & Subsystems/Function-Call Generator  sample_time=-1  numberOfIterations=1  DisallowWideOutput=off
  Function-Call Split : FunctionCallSplit  NumOutputPorts=2
  Function-Call Split1 : FunctionCallSplit  NumOutputPorts=2
  incr_cnt_tmp_mux : Subsystem  TreatAsAtomicUnit=on
      settings: RTWSystemCode=Inline
  parse_cnt_tmp_mux : Subsystem  TreatAsAtomicUnit=on
      settings: RTWSystemCode=Inline
  set_tmp_mux : Subsystem
  wires:
  Function-Call Generator/1 -> Function-Call Split/1
  Function-Call Split/1 -> parse_cnt_tmp_mux/Trigger
  Function-Call Split1/2 -> incr_cnt_tmp_mux/Trigger
  Function-Call Split1/1 -> set_tmp_mux/Trigger
  Function-Call Split/2 -> Function-Call Split1/1

== system npc_controller/IDLE_AND_TIMER/codegen/IDLE/idle_task1/watchdog ==
  note: Note add MLE
  Action Port : ActionPort  ActionPortLabel=case [ 0 ]:
  Watchdog : c281xlib/Watchdog  resetsrc=Specify via dialog  sample=-1
      settings: SourceProductBaseCode=TIC2000

== system npc_controller/IDLE_AND_TIMER/codegen/INITIALIZATION/clb/System Initialize1 ==

== system npc_controller/IDLE_AND_TIMER/codegen/INITIALIZATION/clb/System Initialize2 ==

== system npc_controller/IDLE_AND_TIMER/codegen/INITIALIZATION/clb/System Initialize8 ==

== system npc_controller/IDLE_AND_TIMER/codegen/INITIALIZATION/epwm/System Initialize3 ==

== system npc_controller/IDLE_AND_TIMER/codegen/INITIALIZATION/epwm1/System Initialize1 ==

== system npc_controller/IDLE_AND_TIMER/codegen/INITIALIZATION/epwm1/System Initialize3 ==

== system npc_controller/IDLE_AND_TIMER/codegen/INITIALIZATION/outputxbar/System Initialize1 ==

== system npc_controller/IDLE_AND_TIMER/codegen/INITIALIZATION/outputxbar/System Initialize2 ==

== system npc_controller/IDLE_AND_TIMER/codegen/INITIALIZATION/outputxbar/System Initialize3 ==

== system npc_controller/IDLE_AND_TIMER/codegen/INITIALIZATION/outputxbar/System Initialize4 ==

== system npc_controller/IDLE_AND_TIMER/codegen/INITIALIZATION/outputxbar/System Initialize5 ==

== system npc_controller/IDLE_AND_TIMER/codegen/INITIALIZATION/outputxbar/System Initialize6 ==

== system npc_controller/IDLE_AND_TIMER/codegen/INITIALIZATION/outputxbar/System Initialize7 ==

== system npc_controller/IDLE_AND_TIMER/codegen/TIMER_100MS/incr_cnt/inc ==
  Action Port : ActionPort  ActionPortLabel=else
  Add : Sum
  Constant : Constant  OutDataTypeStr=uint16
  Data Store Read : DataStoreRead  DataStoreName=cnt_poll_can_msg  IndexOptions=Index vector (dialog)  Indices=1  OutputSizes=1
  Data Store Write : DataStoreWrite  DataStoreName=cnt_poll_can_msg  IndexOptions=Index vector (dialog)  Indices=1  OutputSizes=1
  wires:
  Add/1 -> Data Store Write/1
  Data Store Read/1 -> Add/1
  Constant/1 -> Add/2

== system npc_controller/IDLE_AND_TIMER/codegen/TIMER_100MS/incr_cnt/reset ==
  Action Port : ActionPort  ActionPortLabel=if(u1 > 10)
  Constant : Constant  Value=0  OutDataTypeStr=uint16
  Data Store Write : DataStoreWrite  DataStoreName=cnt_poll_can_msg  IndexOptions=Index vector (dialog)  Indices=1  OutputSizes=1
  wires:
  Constant/1 -> Data Store Write/1

== system npc_controller/IDLE_AND_TIMER/codegen/TIMER_1MS/codegen/periodic_timer1 ==
  note: Note:
      |  - Worst error of tfv is timer interval (1ms) + twice the execution of supervisory loop
      |  - Effective max count is 65.536 = 2e16*1e-3
  Add : Sum  Commented=on
  Add1 : Sum
  Constant : Constant  Commented=on  OutDataTypeStr=uint16
  Constant1 : Constant  OutDataTypeStr=uint16
  Data Store Read : DataStoreRead  Commented=on  DataStoreName=cnt_1ms  IndexOptions=Index vector (dialog)  Indices=1  OutputSizes=1
  Data Store Read1 : DataStoreRead  DataStoreName=cnt_1ms  IndexOptions=Index vector (dialog)  Indices=1  OutputSizes=1
  Data Store Write : DataStoreWrite  Commented=on  DataStoreName=cnt_1ms  IndexOptions=Index vector (dialog)  Indices=1  OutputSizes=1
  Data Store Write1 : DataStoreWrite  DataStoreName=cnt_1ms  IndexOptions=Index vector (dialog)  Indices=1  OutputSizes=1
  Rate Transition2 : RateTransition
  Rate Transition3 : RateTransition
  wires:
  Constant/1 -> Add/2
  Add/1 -> Data Store Write/1
  Data Store Read/1 -> Add/1
  Rate Transition3/1 -> Add1/1
  Rate Transition2/1 -> Data Store Write1/1
  Data Store Read1/1 -> Rate Transition3/1
  Add1/1 -> Rate Transition2/1
  Constant1/1 -> Add1/2

== system npc_controller/CONTROL/CONTROL/false/CLA_CONTROL/CONTROL/IIR Filter1 ==
  note: prev 0.98
  x[n] : Inport
  1 - Lambda : Gain  Gain=1-0.9996  ParamDataTypeStr=single  OutDataTypeStr=single
  Delay : Delay  DelayLength=1  StateName=vmid_delay2  StateMustResolveToSignalObject=on
  Delay1 : Delay  DelayLength=1  StateName=vmid_delay1  StateMustResolveToSignalObject=on
  Lambda : Gain  Gain=0.9996  ParamDataTypeStr=single  OutDataTypeStr=single
  Sum : Sum  Inputs=|++  AccumDataTypeStr=single  OutDataTypeStr=single
  y[n] : Outport
  wires:
  Delay/1 -> Lambda/1
  Lambda/1 -> Sum/2
  Sum/1 -> y[n]/1, Delay/1
  1 - Lambda/1 -> Sum/1
  x[n]/1 -> Delay1/1
  Delay1/1 -> 1 - Lambda/1

== system npc_controller/CONTROL/CONTROL/false/CLA_CONTROL/CONTROL/IIR Filter3 ==
  note: prev 0.98
  x[n] : Inport
  1 - Lambda : Gain  Gain=1-0.9996  ParamDataTypeStr=single  OutDataTypeStr=single
  Delay : Delay  DelayLength=1  StateName=vbulk_delay2  StateMustResolveToSignalObject=on
  Delay1 : Delay  DelayLength=1  StateName=vbulk_delay1  StateMustResolveToSignalObject=on
  Lambda : Gain  Gain=0.9996  ParamDataTypeStr=single  OutDataTypeStr=single
  Sum : Sum  Inputs=|++  AccumDataTypeStr=single  OutDataTypeStr=single
  y[n] : Outport
  wires:
  Delay/1 -> Lambda/1
  Lambda/1 -> Sum/2
  Sum/1 -> y[n]/1, Delay/1
  1 - Lambda/1 -> Sum/1
  x[n]/1 -> Delay1/1
  Delay1/1 -> 1 - Lambda/1

== system npc_controller/CONTROL/CONTROL/false/CLA_CONTROL/CONTROL/If Action Subsystem ==
  In1 : Inport
  Action Port : ActionPort  ActionPortLabel=if(u1 == 1)
  Out1 : Outport
  wires:
  In1/1 -> Out1/1

== system npc_controller/CONTROL/CONTROL/false/CLA_CONTROL/CONTROL/If Action Subsystem1 ==
  In1 : Inport
  Action Port : ActionPort  ActionPortLabel=else
  Out1 : Outport
  wires:
  In1/1 -> Out1/1

== system npc_controller/CONTROL/CONTROL/false/CLA_CONTROL/CONTROL/Subsystem1 ==
  note: Note:
      | pol_pha
      | 0 - pos
      | 1 - neg
  iLref : Inport
  vbal_coef : Inport  Port=2
  pol : Inport  Port=3
  AND4 : Logic  Operator=NAND  IconShape=distinctive  AllPortsSameDT=off  OutDataTypeStr=boolean
  AND5 : Logic  IconShape=distinctive  AllPortsSameDT=off  OutDataTypeStr=boolean
  Add : Sum  AccumDataTypeStr=single  OutDataTypeStr=single
  Constant4 : Constant  Value=2  OutDataTypeStr=single  SampleTime=-1
  From3 : From  Commented=on  GotoTag=iLref
  From4 : From  Commented=on  GotoTag=iLref_pos
  From5 : From  Commented=on  GotoTag=iLref_neg
  From52 : From  Commented=on  GotoTag=vbal_coef_top
  From53 : From  Commented=on  GotoTag=vbal_coef_bot
  Mux : Mux  Commented=on  Inputs=3
  Mux1 : Mux  Commented=on  Inputs=2
  Product{4..5,10..11} (4 alike) : Product  OutDataTypeStr=single
  Scope3 : Scope  Commented=on  NumInputPorts=2
  delVdc5 : Sum  Inputs=|+-  AccumDataTypeStr=single  OutDataTypeStr=single
  iLref_vbal : Outport
  wires:
  Mux/1 -> Scope3/2
  Mux1/1 -> Scope3/1
  From52/1 -> Mux1/1
  From53/1 -> Mux1/2
  From5/1 -> Mux/3
  From4/1 -> Mux/2
  From3/1 -> Mux/1
  pol/1 -> [pol]
  Add/1 -> iLref_vbal/1
  iLref/1 -> [iLref]
  vbal_coef/1 -> [vbal_coef_top]
  [vbal_coef_top] -> delVdc5/2
  Constant4/1 -> delVdc5/1
  delVdc5/1 -> [vbal_coef_bot]
  [iLref] -> AND5/1, Product11/1
  Product5/1 -> Add/2
  [iLref_pos] -> Product4/1
  [vbal_coef_top] -> Product4/2
  [iLref_neg] -> Product5/1
  AND4/1 -> Product10/2
  Product4/1 -> Add/1
  Product10/1 -> [iLref_pos]
  [pol] -> AND4/2
  [vbal_coef_bot] -> Product5/2
  [iLref] -> AND4/1, Product10/1
  AND5/1 -> Product11/2
  [pol] -> AND5/2
  Product11/1 -> [iLref_neg]
